simulink model "test"  (R2015a)
settings: Solver=ode45  StartTime=0.0  StopTime=1500  RelTol=1e-3
values from neighbouring files (symbols this model uses):
  EbNo = [0:1:18]    [tes2t.m]
libraries: commdigbbndfm2 x2, commchan3 x1, commrandsrc2 x1, commsink2 x1, commutil2 x1, commrflib2 x1
settings Model: Creator=francisco  LastModifiedBy=francisco

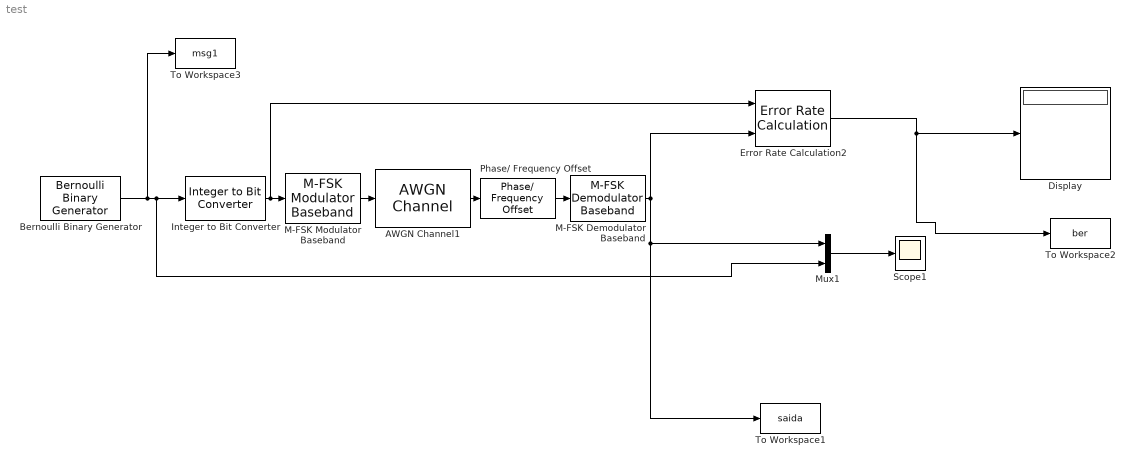
== system test ==
  AWGN Channel1 : commchan3/AWGN Channel  InputProcessing=Columns as channels (frame based)  seed=67  noiseMode="Signal to noise ratio  (Eb/No)"  EbNodB=EbNo  EsNodB=EbNo+10*log10(6)  SNRdB=10  bitsPerSym=1  Ps=1  Tsym=1  variance=1
  Bernoulli Binary Generator : commrandsrc2/Bernoulli Binary Generator  P=0.5  seed=61  Ts=1  frameBased=off  sampPerFrame=1  orient=off  outDataType=double
  Display : Display
  Error Rate Calculation2 : commsink2/Error Rate Calculation  N=0  st_delay=0  cp_mode=Entire frame  subframe=[]  PMode=Port  WsName=ErrorVec  RsMode2=off  stop=off  numErr=100  maxBits=1e6
  Integer to Bit Converter : commutil2/Integer to Bit Converter  nbits=1  signedInputValues=Unsigned  bitOrder=MSB first  outDtype=Inherit via internal rule
  M-FSK Demodulator Baseband : commdigbbndfm2/M-FSK Demodulator Baseband  M=2  OutType=Bit  Dec=Gray  freqSep=200  numSamp=2000  RateOptions=Enforce single-rate processing  outDataType=double
  M-FSK Modulator Baseband : commdigbbndfm2/M-FSK Modulator Baseband  M=2  InType=Bit  Enc=Gray  freqSep=200  phaseType=Continuous  numSamp=2000  RateOptions=Enforce single-rate processing  outDataType=double
  Mux1 : Mux  Inputs=2
  Phase/ Frequency Offset : commrflib2/Phase// Frequency Offset  phaseOffset=90  freqPort=off  freqOffset=0
  Scope1 : Scope
      settings: SaveName=ScopeData2  Decimation=100
  To Workspace1 : ToWorkspace  VariableName=saida  SaveFormat=Timeseries  SampleTime=-1
  To Workspace2 : ToWorkspace  VariableName=ber  SampleTime=-1
      settings: MaxDataPoints=1  Save2DSignal=2-D array (concatenate along first dimension)
  To Workspace3 : ToWorkspace  VariableName=msg1  SaveFormat=Timeseries  SampleTime=-1
  wires:
  Mux1/1 -> Scope1/1
  M-FSK Modulator Baseband/1 -> AWGN Channel1/1
  AWGN Channel1/1 -> Phase/ Frequency Offset/1
  M-FSK Demodulator Baseband/1 -> Mux1/1, To Workspace1/1, Error Rate Calculation2/2
  Bernoulli Binary Generator/1 -> To Workspace3/1, Integer to Bit Converter/1, Mux1/2
  Error Rate Calculation2/1 -> To Workspace2/1, Display/1
  Integer to Bit Converter/1 -> Error Rate Calculation2/1, M-FSK Modulator Baseband/1
  Phase/ Frequency Offset/1 -> M-FSK Demodulator Baseband/1
